simulink model "MotorControlRL"  (R2022b)
settings: Solver=VariableStepAuto  StartTime=0.0  StopTime=2000  RelTol=1e-3
model workspace (MAT data in the model file):
  J = 0.0008241
  Kb = 0.085711
  Kt = 0.085711
  La = 0.0001129
  Ra = 1.86
  RatedSpeed = 1500
  RequiredSpeed = 300
  b = 0.00382
undefined symbols (not defined in the file): DiscIntNeverNeededParam
libraries: simulink x1, dspstat3 x1, rllib x1
settings Model: Creator=MERUGA KISHAN BALAJI  LastModifiedBy=MERUGA KISHAN BALAJI
settings DebuggingCC: ParameterOverflowMsg=none  ParameterUnderflowMsg=error  ParameterPrecisionLossMsg=none

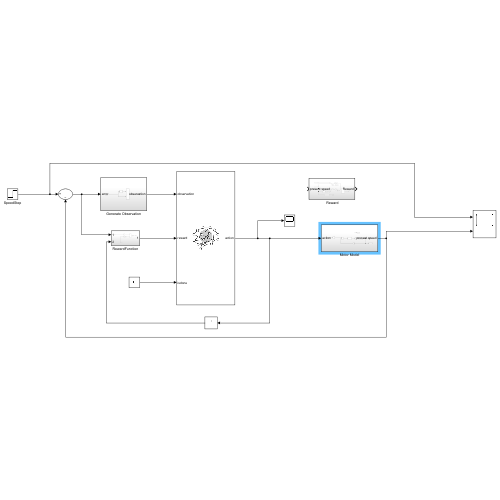
[thumbnail: Simulink's stored preview of the top-level diagram]
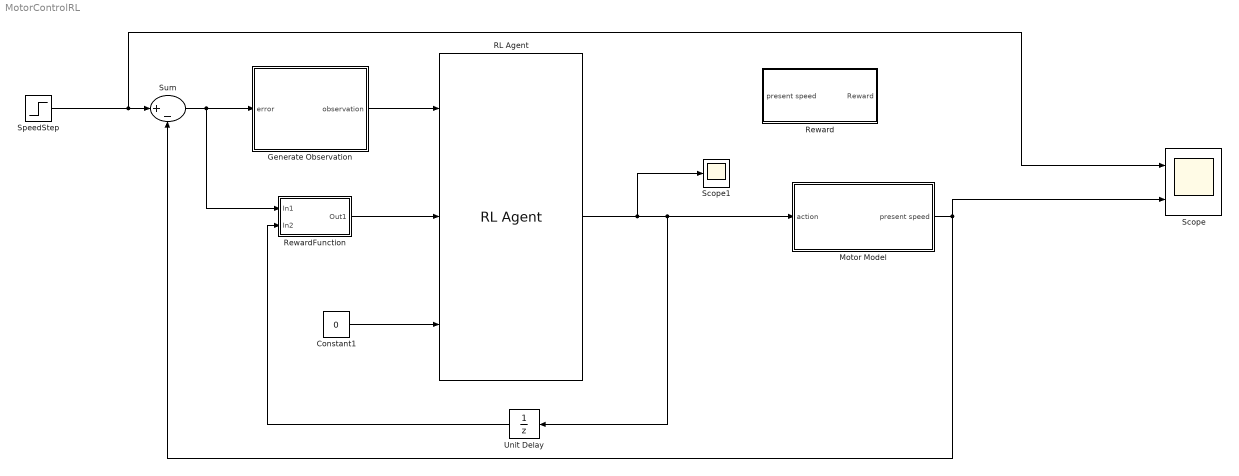
== system MotorControlRL ==
  " Reward" : Subsystem
  Constant1 : Constant  Value=0
  Generate Observation : Subsystem
  Motor Model : Subsystem
  RL Agent : rllib/RL Agent  Agent=agent  ExternalActionAsInput=off  ProvideLastAction=off  ProvideCumRwd=off  TreatAsDirectFeedthrough=on  UseStrictObservationDataTypes=off
  RewardFunction : Subsystem
  Scope : Scope  NumInputPorts=2
  Scope1 : Scope
  SpeedStep : Step  Time=1000  Before=600  After=900  SampleTime=0
  Sum : Sum  Inputs=|+-
  Unit Delay : UnitDelay  SampleTime=-1  HasFrameUpgradeWarning=on
  wires:
  SpeedStep/1 -> Sum/1, Scope/1
  Sum/1 -> RewardFunction/1(In1), Generate Observation/1(error)
  Generate Observation/1(observation) -> RL Agent/1
  RL Agent/1 -> Unit Delay/1, Motor Model/1(action), Scope1/1
  Constant1/1 -> RL Agent/3
  Motor Model/1(present speed) -> Sum/2, Scope/2
  Unit Delay/1 -> RewardFunction/2(In2)
  RewardFunction/1(Out1) -> RL Agent/2

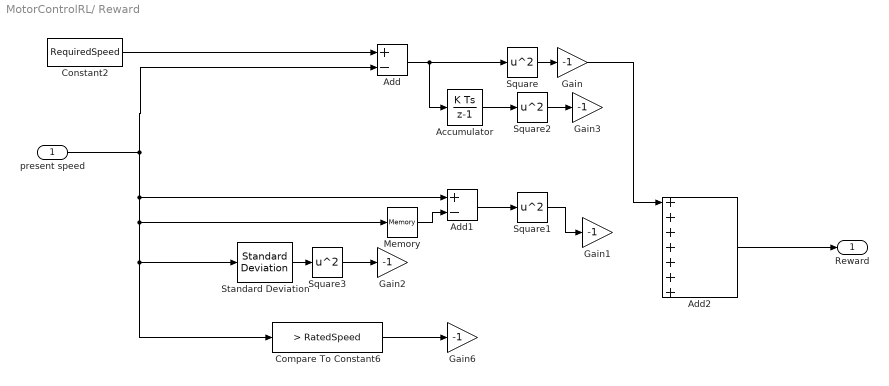
== system MotorControlRL/ Reward ==
  present speed : Inport
  Accumulator : DiscreteIntegrator  gainval=1  SampleTime=-1  ICPrevOutput=DiscIntNeverNeededParam  ICPrevScaledInput=DiscIntNeverNeededParam
  Add : Sum  Inputs=+-
  Add1 : Sum  Inputs=+-
  Add2 : Sum  Inputs=+++++++
  Compare To Constant6 : simulink/Logic and Bit Operations/Compare To Constant  relop=>  const=RatedSpeed  OutDataTypeStr=boolean
  Constant2 : Constant  Value=RequiredSpeed
  Gain{,1..3,6} (5 alike) : Gain  Gain=-1
  Memory : Memory
  Square{,1..3} (4 alike) : Math  Operator=square  SignedPower=on  RndMeth=Zero
  Standard Deviation : dspstat3/Standard Deviation  run=off  directionMode=Entire input  dimension=1  InputProcessing=Columns as channels (frame based)  reset_popup=None  roiEnable=off  roiType=Rectangles  roiPortion=Entire ROI  roiOutput=Individual statistics for each ROI  roiFlag=off
  Reward : Outport
  wires:
  present speed/1 -> Memory/1, Compare To Constant6/1, Standard Deviation/1, Add1/1, Add/2
  Compare To Constant6/1 -> Gain6/1
  Add1/1 -> Square1/1
  Memory/1 -> Add1/2
  Constant2/1 -> Add/1
  Add2/1 -> Reward/1
  Add/1 -> Accumulator/1, Square/1
  Gain/1 -> Add2/1
  Square1/1 -> Gain1/1
  Square/1 -> Gain/1
  Accumulator/1 -> Square2/1
  Square2/1 -> Gain3/1
  Standard Deviation/1 -> Square3/1
  Square3/1 -> Gain2/1

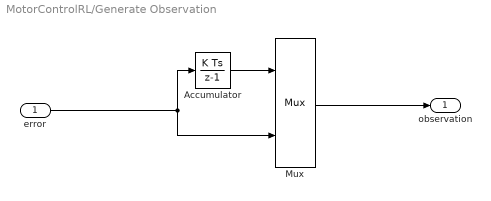
== system MotorControlRL/Generate Observation ==
  error : Inport
  Accumulator : DiscreteIntegrator  gainval=1  SampleTime=-1  ICPrevOutput=DiscIntNeverNeededParam  ICPrevScaledInput=DiscIntNeverNeededParam
  Mux : Mux  Inputs=2
  observation : Outport
  wires:
  error/1 -> Accumulator/1, Mux/2
  Accumulator/1 -> Mux/1
  Mux/1 -> observation/1

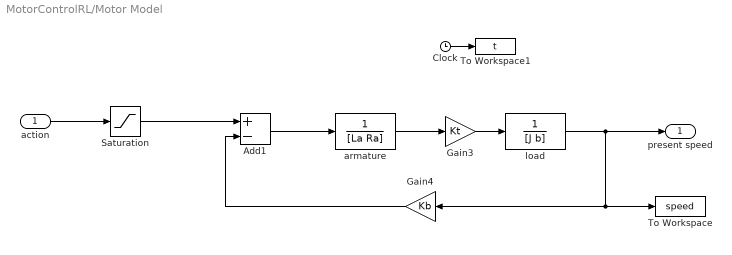
== system MotorControlRL/Motor Model ==
  action : Inport
  Add1 : Sum  Inputs=+-
  Clock : Clock
  Gain3 : Gain  Gain=Kt
  Gain4 : Gain  Gain=Kb
  Saturation : Saturate  UpperLimit=255  LowerLimit=-255
  To Workspace : ToWorkspace  VariableName=speed  SaveFormat=Timeseries  SampleTime=-1
  To Workspace1 : ToWorkspace  VariableName=t  SaveFormat=Timeseries
  armature : TransferFcn  Denominator=[La Ra]
  load : TransferFcn  Denominator=[J b]
  present speed : Outport
  wires:
  Gain4/1 -> Add1/2
  armature/1 -> Gain3/1
  Add1/1 -> armature/1
  Gain3/1 -> load/1
  Clock/1 -> To Workspace1/1
  load/1 -> To Workspace/1, Gain4/1, present speed/1
  Saturation/1 -> Add1/1
  action/1 -> Saturation/1

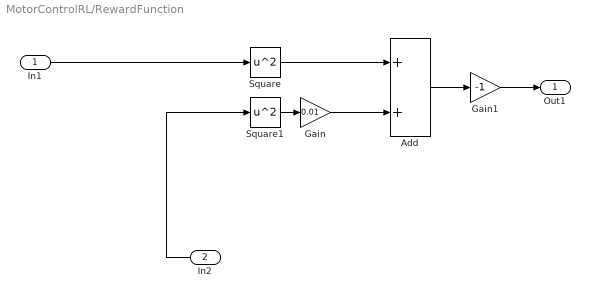
== system MotorControlRL/RewardFunction ==
  In1 : Inport
  In2 : Inport  Port=2
  Add : Sum
  Gain : Gain  Gain=0.01
  Gain1 : Gain  Gain=-1
  Square : Math  Operator=square  SignedPower=on  RndMeth=Zero
  Square1 : Math  Operator=square  SignedPower=on  RndMeth=Zero
  Out1 : Outport
  wires:
  Square1/1 -> Gain/1
  Add/1 -> Gain1/1
  In1/1 -> Square/1
  Square/1 -> Add/1
  Gain/1 -> Add/2
  In2/1 -> Square1/1
  Gain1/1 -> Out1/1
